simulink model "cascaded_controller"  (R2025b)
settings: Solver=FixedStepAuto  StartTime=0.0  StopTime=10.0  RelTol=1e-3  SampleTimeConstraint=Specified
undefined symbols (not defined in the file): dt_control
libraries: ros2lib x3
settings Model: Creator=vulcangrip  LastModifiedBy=vulcangrip
settings OptimizationCC: DefaultParameterBehavior=Inlined  EnhancedBackFolding=on  PassReuseOutputArgsAs=Individual arguments  ZeroExternalMemoryAtStartup=off  ZeroInternalMemoryAtStartup=off  MaxStackSize=64  OptimizeBlockOrder=speed  DifferentSizesBufferReuse=on  OptimizationCustomize=off  EfficientTunableParamExpr=on
settings DebuggingCC: ParameterTunabilityLossMsg=error
settings HardwareCC: ProdBitPerLong=64.0  ProdLargestAtomicInteger=LongLong  ProdLargestAtomicFloat=Double  ProdLongLongMode=on  ProdHWDeviceType=ARM Compatible->ARM Cortex-A (64-bit)
settings SFSimCC: MATLABDynamicMemAlloc=off  SimTargetLang=C++  SimDLTargetLibrary=mkl-dnn
settings RTWCC: SystemTargetFile=ert.tlc  HardwareBoard=Robot Operating System 2 (ROS 2)  TLCOptions="-aInlineSetEventsForThisBaseRateFcn=TLC_FALSE -aSuppressMultiTaskScheduler=TLC_FALSE  -aRateBasedStepFcn=0"  GenCodeOnly=on  TemplateMakefile=ert_default_tmf  Toolchain=Colcon Tools  TargetLang=C++  Description=Embedded Coder
settings CodeAppCC: ForceParamTrailComments=on  IgnoreCustomStorageClasses=off  OperatorAnnotations=on  SimulinkDataObjDesc=on  SFDataObjDesc=on  InsertBlockDesc=on
settings ERTTargetCC: ExtModeTransport=2.0  ExtModeStaticAlloc=on  ExtModeAutomaticAllocSize=off  ExtModeMexFile=ext_xcp  ExtModeIntrfLevel=Level2 - Open  RootIOFormat=Structure reference  TargetLangStandard=C++11 (ISO)  CodeInterfacePackaging=C++ class  SupportVariableSizeSignals=on

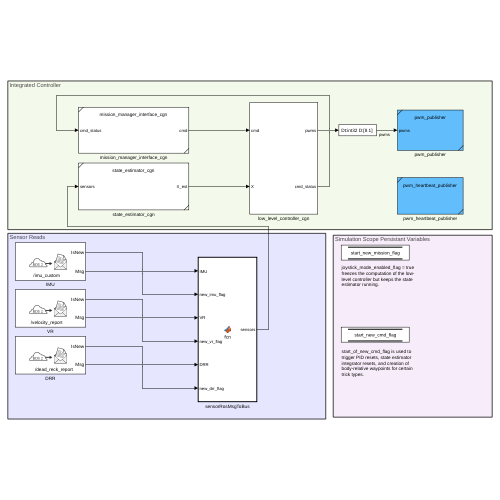
[thumbnail: Simulink's stored preview of the top-level diagram]
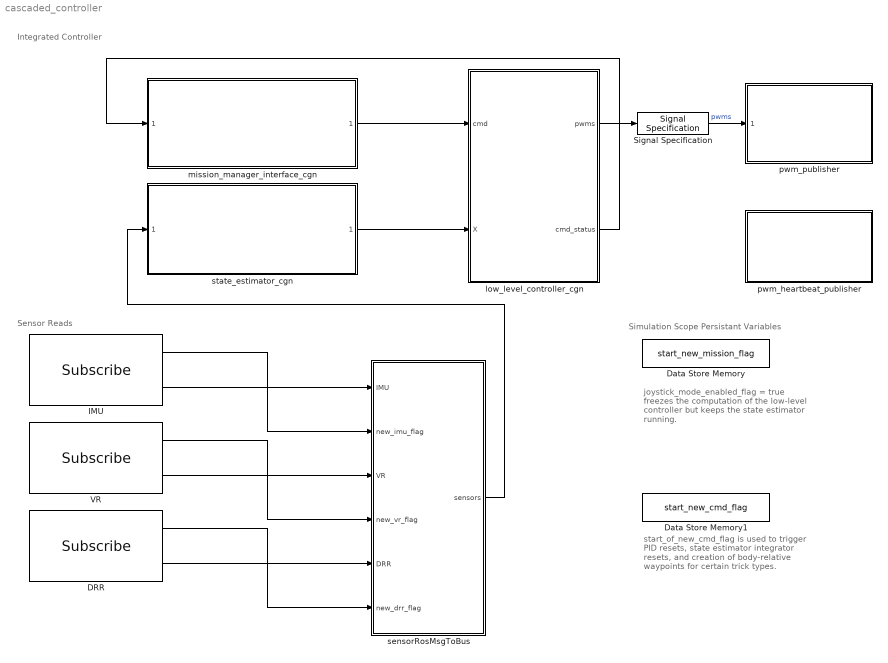
== system cascaded_controller ==
  note: Integrated Controller
  note: Simulation Scope Persistant Variables
  note: joystick_mode_enabled_flag = true freezes the computation of the low-level controller but keeps the state estimator running.
  note: start_of_new_cmd_flag is used to trigger PID resets, state estimator integrator resets, and creation of body-relative waypoints for certain trick types.
  note: Sensor Reads
  DRR : ros2lib/Subscribe  topicSource=Select from ROS network  topic=/dead_reck_report  messageType=custom_interfaces/DRR  sampleTime=-1  QOSHistory=Keep last  QOSDepth=10  QOSReliability=Reliable  QOSDurability=Volatile  QOSDeadline=Inf  QOSLifespan=Inf  QOSLiveliness=Automatic  QOSLeaseDuration=Inf  QOSAvoidROSNamespaceConventions=off
  Data Store Memory : DataStoreMemory  DataStoreName=start_new_mission_flag  WriteAfterWriteMsg=warning  InitialValue=initial_joystick_mode_enabled_flag  ShowAdditionalParam=off  OutDataTypeStr=boolean
  Data Store Memory1 : DataStoreMemory  DataStoreName=start_new_cmd_flag  WriteAfterWriteMsg=warning  InitialValue=false  ShowAdditionalParam=off  OutDataTypeStr=boolean
  IMU : ros2lib/Subscribe  topicSource=Specify your own  topic=/imu_custom  messageType=custom_interfaces/Imu  sampleTime=1/100  QOSHistory=Keep last  QOSDepth=10  QOSReliability=Reliable  QOSDurability=Volatile  QOSDeadline=Inf  QOSLifespan=Inf  QOSLiveliness=Automatic  QOSLeaseDuration=Inf  QOSAvoidROSNamespaceConventions=off
  Signal Specification : SignalSpecification  OutDataTypeStr=int32  Dimensions=[8 1]
  VR : ros2lib/Subscribe  topicSource=Select from ROS network  topic=/velocity_report  messageType=custom_interfaces/VR  sampleTime=-1  QOSHistory=Keep last  QOSDepth=10  QOSReliability=Reliable  QOSDurability=Volatile  QOSDeadline=Inf  QOSLifespan=Inf  QOSLiveliness=Automatic  QOSLeaseDuration=Inf  QOSAvoidROSNamespaceConventions=off
  low_level_controller_cgn : Subsystem
  mission_manager_interface_cgn : Subsystem  ReferencedSubsystem=mission_manager_interface_cgn
  pwm_heartbeat_publisher : Subsystem  ReferencedSubsystem=pwm_heartbeat_publisher
  pwm_publisher : Subsystem  ReferencedSubsystem=pwm_publisher
  sensorRosMsgToBus : MATLAB Function  TreatAsAtomicUnit=on
  state_estimator_cgn : Subsystem  ReferencedSubsystem=state_estimator_cgn
  wires:
  VR/2 -> sensorRosMsgToBus/3(VR)
  low_level_controller_cgn/1(pwms) -> Signal Specification/1
  DRR/1 -> sensorRosMsgToBus/6(new_drr_flag)
  VR/1 -> sensorRosMsgToBus/4(new_vr_flag)
  low_level_controller_cgn/2(cmd_status) -> mission_manager_interface_cgn/1
  state_estimator_cgn/1 -> low_level_controller_cgn/2(X)
  IMU/1 -> sensorRosMsgToBus/2(new_imu_flag)
  DRR/2 -> sensorRosMsgToBus/5(DRR)
  sensorRosMsgToBus/1(sensors) -> state_estimator_cgn/1
  mission_manager_interface_cgn/1 -> low_level_controller_cgn/1(cmd)
  Signal Specification/1 -> pwm_publisher/1  "pwms"
  IMU/2 -> sensorRosMsgToBus/1(IMU)

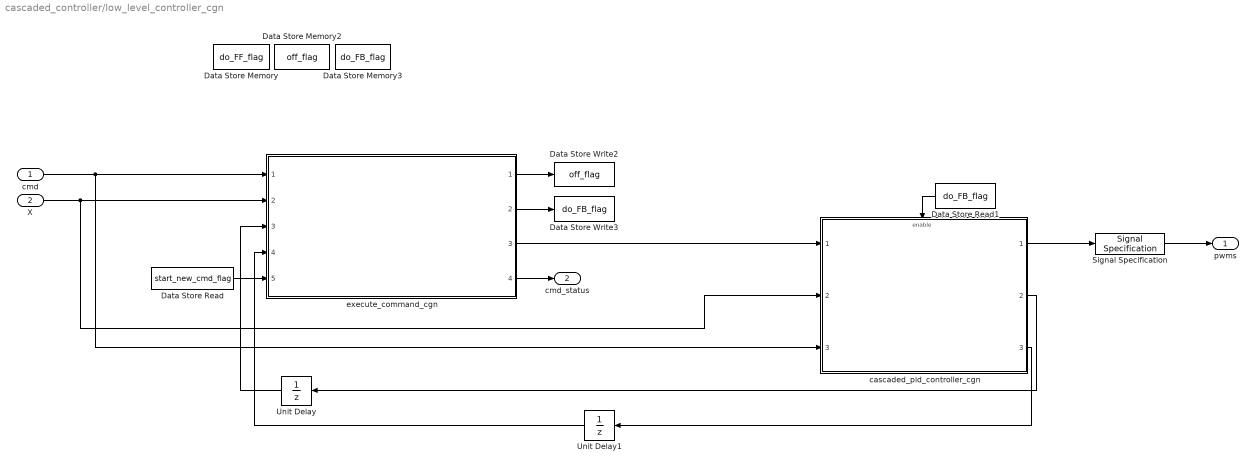
== system cascaded_controller/low_level_controller_cgn ==
  cmd : Inport  OutDataTypeStr=Bus: cmd_bus  SampleTime=dt_control
      settings: VarSizeSig=Yes
  X : Inport  Port=2  SampleTime=dt_control
  Data Store Memory : DataStoreMemory  DataStoreName=do_FF_flag  WriteAfterWriteMsg=warning  ShowAdditionalParam=off
  Data Store Memory2 : DataStoreMemory  DataStoreName=off_flag  WriteAfterWriteMsg=warning  ShowAdditionalParam=off
  Data Store Memory3 : DataStoreMemory  DataStoreName=do_FB_flag  WriteAfterWriteMsg=warning  ShowAdditionalParam=off
  Data Store Read : DataStoreRead  DataStoreName=start_new_cmd_flag  IndexOptions=Index vector (dialog)  Indices=1  OutputSizes=1
  Data Store Read1 : DataStoreRead  DataStoreName=do_FB_flag  IndexOptions=Index vector (dialog)  Indices=1  OutputSizes=1
  Data Store Write2 : DataStoreWrite  DataStoreName=off_flag  IndexOptions=Index vector (dialog)  Indices=1  OutputSizes=1
  Data Store Write3 : DataStoreWrite  DataStoreName=do_FB_flag  IndexOptions=Index vector (dialog)  Indices=1  OutputSizes=1
  Signal Specification : SignalSpecification  OutDataTypeStr=int32
  Unit Delay : UnitDelay  SampleTime=dt_control  HasFrameUpgradeWarning=on
  Unit Delay1 : UnitDelay  SampleTime=dt_control  HasFrameUpgradeWarning=on
  cascaded_pid_controller_cgn : Subsystem  ReferencedSubsystem=cascaded_pid_controller_cgn
  execute_command_cgn : Subsystem  ReferencedSubsystem=execute_command_cgn
  pwms : Outport
  cmd_status : Outport  Port=2  SampleTime=dt_control
  wires:
  Unit Delay1/1 -> execute_command_cgn/4
  cmd/1 -> cascaded_pid_controller_cgn/3, execute_command_cgn/1
  execute_command_cgn/4 -> cmd_status/1
  execute_command_cgn/2 -> Data Store Write3/1
  execute_command_cgn/3 -> cascaded_pid_controller_cgn/1
  execute_command_cgn/1 -> Data Store Write2/1
  cascaded_pid_controller_cgn/2 -> Unit Delay/1
  cascaded_pid_controller_cgn/3 -> Unit Delay1/1
  X/1 -> cascaded_pid_controller_cgn/2, execute_command_cgn/2
  Unit Delay/1 -> execute_command_cgn/3
  Signal Specification/1 -> pwms/1
  Data Store Read1/1 -> cascaded_pid_controller_cgn/Enable
  cascaded_pid_controller_cgn/1 -> Signal Specification/1
  Data Store Read/1 -> execute_command_cgn/5

== matlab function cascaded_controller/sensorRosMsgToBus ==
  data: IMU input Bus: SL_Bus_custom_interfaces_Imu; new_imu_flag input; sensors output Bus: sensor_bus; VR input Bus: SL_Bus_custom_interfaces_VR; new_vr_flag input; DRR input Bus: SL_Bus_custom_interfaces_DRR size=[1,1]; new_drr_flag input
function sensors = fcn(IMU, new_imu_flag, VR, new_vr_flag, DRR, new_drr_flag)

sensors = sensorRosMsgToBus(IMU, new_imu_flag, VR, new_vr_flag, DRR, new_drr_flag);
